simulink model "ambiente_teste"  (R2021b)
settings: Solver=VariableStepAuto  StartTime=0.0  StopTime=5  RelTol=1e-3
values from neighbouring files (symbols this model uses):
  a = 2*wn*zeta    [find_tf.m]    (also in identifica.mat = 14.2666203069; setup_lab_ip01_2.m = 1; teste.mat = 1)
  b = (wn^2)/C    [find_tf.m]    (also in identifica.mat = 1.26932415875; setup_lab_ip01_2.m = 1; teste.mat = 1)
  T = Td/32    [find_tf.m]
  VMAX_AMP = 12    [identifica.mat]    (also in setup_ip01_2_configuration.m = 4.16; teste.mat)
settings Model: Creator=Gabriel Vieira  LastModifiedBy=Gabriel Vieira

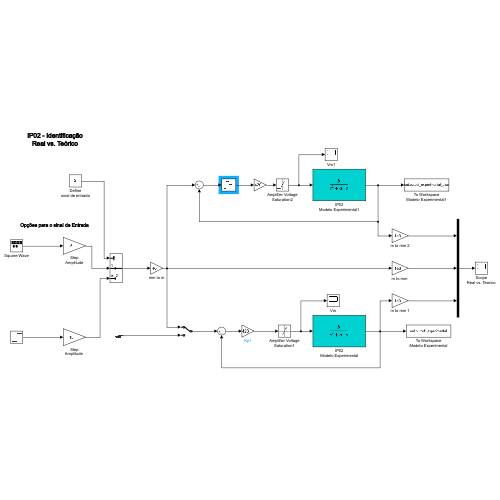
[thumbnail: Simulink's stored preview of the top-level diagram]
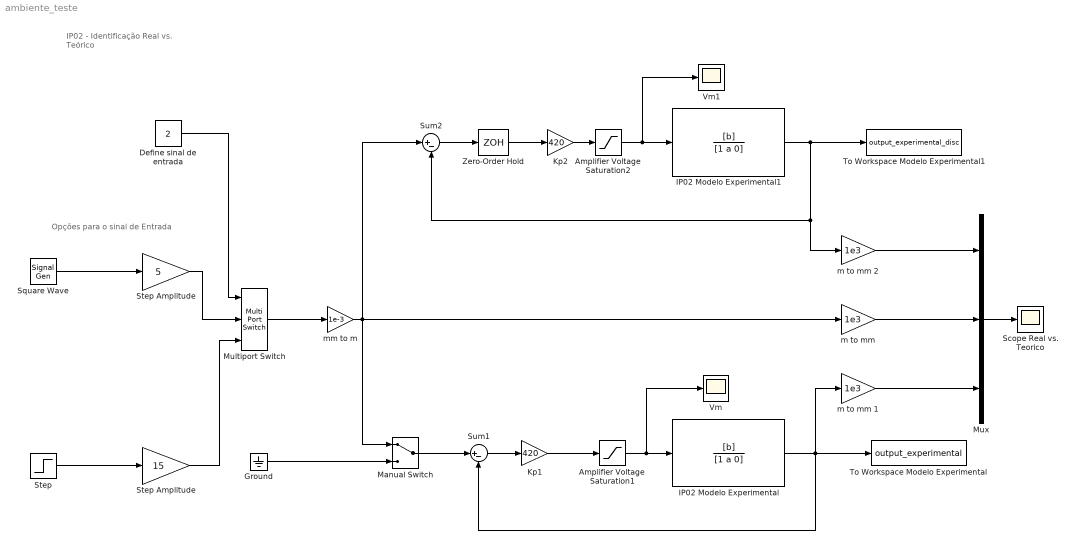
== system ambiente_teste ==
  note: Opções para o sinal de Entrada
  note: IP02 - Identificação
      | Real vs. Teórico
  Amplifier Voltage Saturation1 : Saturate  UpperLimit=VMAX_AMP  LowerLimit=- VMAX_AMP
  Amplifier Voltage Saturation2 : Saturate  UpperLimit=VMAX_AMP  LowerLimit=- VMAX_AMP
  Define sinal de entrada : Constant  Value=2
  Ground : Ground
  IP02 Modelo Experimental : TransferFcn  Numerator=[b]  Denominator=[1 a 0]
  IP02 Modelo Experimental1 : TransferFcn  Numerator=[b]  Denominator=[1 a 0]
  Kp1 : Gain  Gain=420  SaturateOnIntegerOverflow=on  OutDataTypeStr=Inherit: Same as input  ParamDataTypeStr=Inherit: Same as input
  Kp2 : Gain  Gain=420  SaturateOnIntegerOverflow=on  OutDataTypeStr=Inherit: Same as input  ParamDataTypeStr=Inherit: Same as input
  Manual Switch : ManualSwitch
  Multiport Switch : MultiPortSwitch  Inputs=2
  Mux : Mux  Inputs=3
  Scope Real vs. Teorico : Scope
  Square Wave : SignalGenerator  WaveForm=square  Frequency=0.66
  Step : Step  Time=0  SampleTime=0
  Step Amplitude : Gain  Gain=5  SaturateOnIntegerOverflow=on  OutDataTypeStr=Inherit: Same as input  ParamDataTypeStr=Inherit: Same as input
  "Step Amplitude " : Gain  Gain=15  SaturateOnIntegerOverflow=on  OutDataTypeStr=Inherit: Same as input  ParamDataTypeStr=Inherit: Same as input
  Sum1 : Sum  Inputs=|+-  InputSameDT=on  SaturateOnIntegerOverflow=on  OutDataTypeStr=Inherit: Same as first input
  Sum2 : Sum  Inputs=|+-  InputSameDT=on  SaturateOnIntegerOverflow=on  OutDataTypeStr=Inherit: Same as first input
  To Workspace Modelo Experimental : ToWorkspace  VariableName=output_experimental  SaveFormat=Structure With Time  SampleTime=-1
  To Workspace Modelo Experimental1 : ToWorkspace  VariableName=output_experimental_disc  SaveFormat=Structure With Time  SampleTime=-1
  Vm : Scope
  Vm1 : Scope
  Zero-Order Hold : ZeroOrderHold  SampleTime=T
  "m to mm " : Gain  Gain=1e3  SaturateOnIntegerOverflow=on  OutDataTypeStr=Inherit: Same as input  ParamDataTypeStr=Inherit: Same as input
  m to mm 1 : Gain  Gain=1e3  SaturateOnIntegerOverflow=on  OutDataTypeStr=Inherit: Same as input  ParamDataTypeStr=Inherit: Same as input
  m to mm 2 : Gain  Gain=1e3  SaturateOnIntegerOverflow=on  OutDataTypeStr=Inherit: Same as input  ParamDataTypeStr=Inherit: Same as input
  mm to m : Gain  Gain=1e-3
  wires:
  m to mm 1/1 -> Mux/3
  Multiport Switch/1 -> mm to m/1
  Square Wave/1 -> Step Amplitude/1
  Kp1/1 -> Amplifier Voltage Saturation1/1
  Step/1 -> "Step Amplitude "/1
  "Step Amplitude "/1 -> Multiport Switch/3
  Sum1/1 -> Kp1/1
  Amplifier Voltage Saturation1/1 -> Vm/1, IP02 Modelo Experimental/1
  Mux/1 -> Scope Real vs. Teorico/1
  Ground/1 -> Manual Switch/2
  IP02 Modelo Experimental/1 -> To Workspace Modelo Experimental/1, Sum1/2, m to mm 1/1
  Manual Switch/1 -> Sum1/1
  "m to mm "/1 -> Mux/2
  Define sinal de entrada/1 -> Multiport Switch/1
  Step Amplitude/1 -> Multiport Switch/2
  m to mm 2/1 -> Mux/1
  mm to m/1 -> Sum2/1, "m to mm "/1, Manual Switch/1
  IP02 Modelo Experimental1/1 -> Sum2/2, m to mm 2/1, To Workspace Modelo Experimental1/1
  Amplifier Voltage Saturation2/1 -> Vm1/1, IP02 Modelo Experimental1/1
  Kp2/1 -> Amplifier Voltage Saturation2/1
  Sum2/1 -> Zero-Order Hold/1
  Zero-Order Hold/1 -> Kp2/1
